simulink model "PM_fnc16_DevHarness_ExLoad"  (R2022a)
settings: Solver=VariableStepAuto  StartTime=0.0  StopTime=10.0  RelTol=1e-3
settings Model: Creator=306427  LastModifiedBy=306427

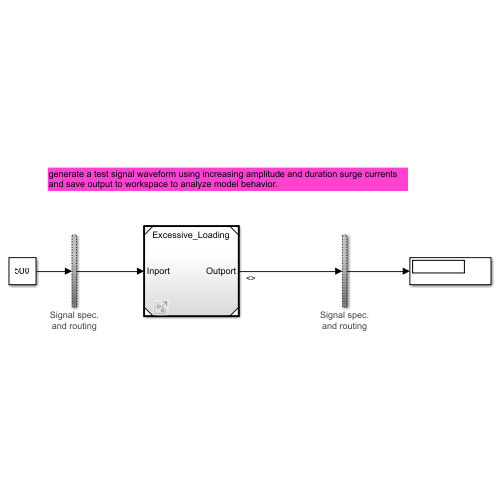
[thumbnail: Simulink's stored preview of the top-level diagram]
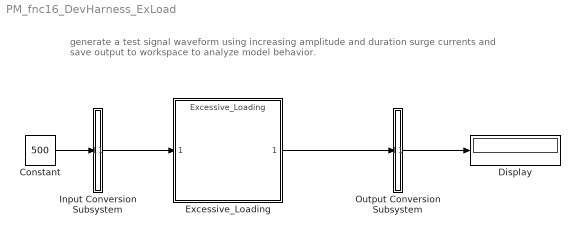
== system PM_fnc16_DevHarness_ExLoad ==
  note: generate a test signal waveform using increasing amplitude and duration surge currents and save output to workspace to analyze model behavior.
  Constant : Constant  Value=500  OutDataTypeStr=uint16
  Display : Display
  Excessive_Loading : ModelReference  ModelNameDialog=Excessive_Loading  SimulationMode=Normal  ModelReferenceVersion=1.9
  Input Conversion Subsystem : Subsystem  Tag=__SLT_ICS__  Description=|
      | Signal spec.
      | and routing
      settings: AttributesFormatString=%<Description>
  Output Conversion Subsystem : Subsystem  Tag=__SLT_OCS__  Description=|
      | Signal spec.
      | and routing
      settings: AttributesFormatString=%<Description>
  wires:
  Constant/1 -> Input Conversion Subsystem/1(Inport_1)
  Output Conversion Subsystem/1(Outport_1) -> Display/1
  Input Conversion Subsystem/1(Outport_1) -> Excessive_Loading/1
  Excessive_Loading/1 -> Output Conversion Subsystem/1(Inport_1)

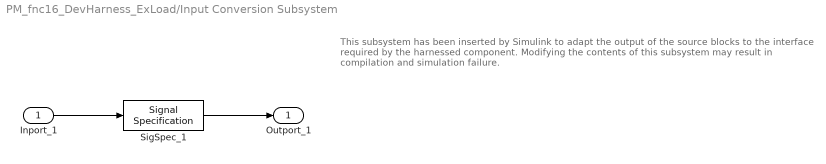
== system PM_fnc16_DevHarness_ExLoad/Input Conversion Subsystem ==
  note: This subsystem has been inserted by Simulink to adapt the output of the source blocks to the interface required by the harnessed component.
      |  Modifying the contents of this subsystem may result in compilation and simulation failure.
  Inport_1 : Inport
  SigSpec_1 : SignalSpecification  OutDataTypeStr=uint16  Dimensions=[1]  SampleTime=[0, 0]
  Outport_1 : Outport
  wires:
  SigSpec_1/1 -> Outport_1/1
  Inport_1/1 -> SigSpec_1/1

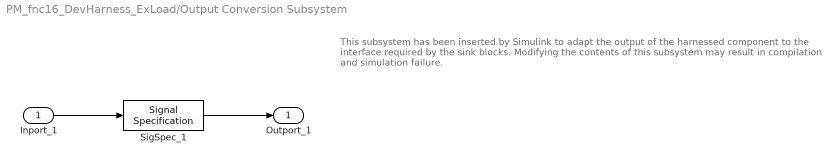
== system PM_fnc16_DevHarness_ExLoad/Output Conversion Subsystem ==
  note: This subsystem has been inserted by Simulink to adapt the output of the harnessed component to the interface required by the sink blocks.
      |  Modifying the contents of this subsystem may result in compilation and simulation failure.
  Inport_1 : Inport
  SigSpec_1 : SignalSpecification  OutDataTypeStr=uint16  Dimensions=[1]
  Outport_1 : Outport
  wires:
  Inport_1/1 -> SigSpec_1/1
  SigSpec_1/1 -> Outport_1/1
